simulink model "untitled"  (R2020b)
(part 3 of 4)

  BodyLSum517/1 -> BodyLSum518/2
  BodyDelay518/1 -> b(518)/1, BodyDelay519/1
  b(518)/1 -> BodyLSum518/1
  BodyLSum518/1 -> BodyLSum519/2
  BodyDelay519/1 -> b(519)/1, BodyDelay520/1
  b(519)/1 -> BodyLSum519/1
  BodyLSum519/1 -> BodyLSum520/2
  BodyDelay520/1 -> b(520)/1, BodyDelay521/1
  b(520)/1 -> BodyLSum520/1
  BodyLSum520/1 -> BodyLSum521/2
  BodyDelay521/1 -> b(521)/1, BodyDelay522/1
  b(521)/1 -> BodyLSum521/1
  BodyLSum521/1 -> BodyLSum522/2
  BodyDelay522/1 -> b(522)/1, BodyDelay523/1
  b(522)/1 -> BodyLSum522/1
  BodyLSum522/1 -> BodyLSum523/2
  BodyDelay523/1 -> b(523)/1, BodyDelay524/1
  b(523)/1 -> BodyLSum523/1
  BodyLSum523/1 -> BodyLSum524/2
  BodyDelay524/1 -> b(524)/1, BodyDelay525/1
  b(524)/1 -> BodyLSum524/1
  BodyLSum524/1 -> BodyLSum525/2
  BodyDelay525/1 -> b(525)/1, BodyDelay526/1
  b(525)/1 -> BodyLSum525/1
  BodyLSum525/1 -> BodyLSum526/2
  BodyDelay526/1 -> b(526)/1, BodyDelay527/1
  b(526)/1 -> BodyLSum526/1
  BodyLSum526/1 -> BodyLSum527/2
  BodyDelay527/1 -> b(527)/1, BodyDelay528/1
  b(527)/1 -> BodyLSum527/1
  BodyLSum527/1 -> BodyLSum528/2
  BodyDelay528/1 -> b(528)/1, BodyDelay529/1
  b(528)/1 -> BodyLSum528/1
  BodyLSum528/1 -> BodyLSum529/2
  BodyDelay529/1 -> b(529)/1, BodyDelay530/1
  b(529)/1 -> BodyLSum529/1
  BodyLSum529/1 -> BodyLSum530/2
  BodyDelay530/1 -> b(530)/1, BodyDelay531/1
  b(530)/1 -> BodyLSum530/1
  BodyLSum530/1 -> BodyLSum531/2
  BodyDelay531/1 -> b(531)/1, BodyDelay532/1
  b(531)/1 -> BodyLSum531/1
  BodyLSum531/1 -> BodyLSum532/2
  BodyDelay532/1 -> b(532)/1, BodyDelay533/1
  b(532)/1 -> BodyLSum532/1
  BodyLSum532/1 -> BodyLSum533/2
  BodyDelay533/1 -> b(533)/1, BodyDelay534/1
  b(533)/1 -> BodyLSum533/1
  BodyLSum533/1 -> BodyLSum534/2
  BodyDelay534/1 -> b(534)/1, BodyDelay535/1
  b(534)/1 -> BodyLSum534/1
  BodyLSum534/1 -> BodyLSum535/2
  BodyDelay535/1 -> b(535)/1, BodyDelay536/1
  b(535)/1 -> BodyLSum535/1
  BodyLSum535/1 -> BodyLSum536/2
  BodyDelay536/1 -> b(536)/1, BodyDelay537/1
  b(536)/1 -> BodyLSum536/1
  BodyLSum536/1 -> BodyLSum537/2
  BodyDelay537/1 -> b(537)/1, BodyDelay538/1
  b(537)/1 -> BodyLSum537/1
  BodyLSum537/1 -> BodyLSum538/2
  BodyDelay538/1 -> b(538)/1, BodyDelay539/1
  b(538)/1 -> BodyLSum538/1
  BodyLSum538/1 -> BodyLSum539/2
  BodyDelay539/1 -> b(539)/1, BodyDelay540/1
  b(539)/1 -> BodyLSum539/1
  BodyLSum539/1 -> BodyLSum540/2
  BodyDelay540/1 -> b(540)/1, BodyDelay541/1
  b(540)/1 -> BodyLSum540/1
  BodyLSum540/1 -> BodyLSum541/2
  BodyDelay541/1 -> b(541)/1, BodyDelay542/1
  b(541)/1 -> BodyLSum541/1
  BodyLSum541/1 -> BodyLSum542/2
  BodyDelay542/1 -> b(542)/1, BodyDelay543/1
  b(542)/1 -> BodyLSum542/1
  BodyLSum542/1 -> BodyLSum543/2
  BodyDelay543/1 -> b(543)/1, BodyDelay544/1
  b(543)/1 -> BodyLSum543/1
  BodyLSum543/1 -> BodyLSum544/2
  BodyDelay544/1 -> b(544)/1, BodyDelay545/1
  b(544)/1 -> BodyLSum544/1
  BodyLSum544/1 -> BodyLSum545/1
  BodyDelay545/1 -> b(545)/1
  b(545)/1 -> BodyLSum545/2
  BodyLSum545/1 -> Output/1
